simulink model "PV_battery"  (R2017b)
settings: Solver=FixedStepDiscrete  StartTime=0.0  StopTime=1  FixedStep=Ts  RelTol=1e-3
InitFcn:
  | Ts=0.000001;
undefined symbols (not defined in the file): DiscIntNeverNeededParam, Ion, Lithium, sigbuilder_block
libraries: powerlib x29, powerlib_meascontrol x2, simulink x2, fuzblock x1, electricdrivelib x1, re_lib x1
settings Model: Creator=Aria  LastModifiedBy=Asus
settings CodeAppCC: StateflowObjectComments=on
settings SimscapeCC: SimscapeNormalizeSystem=off

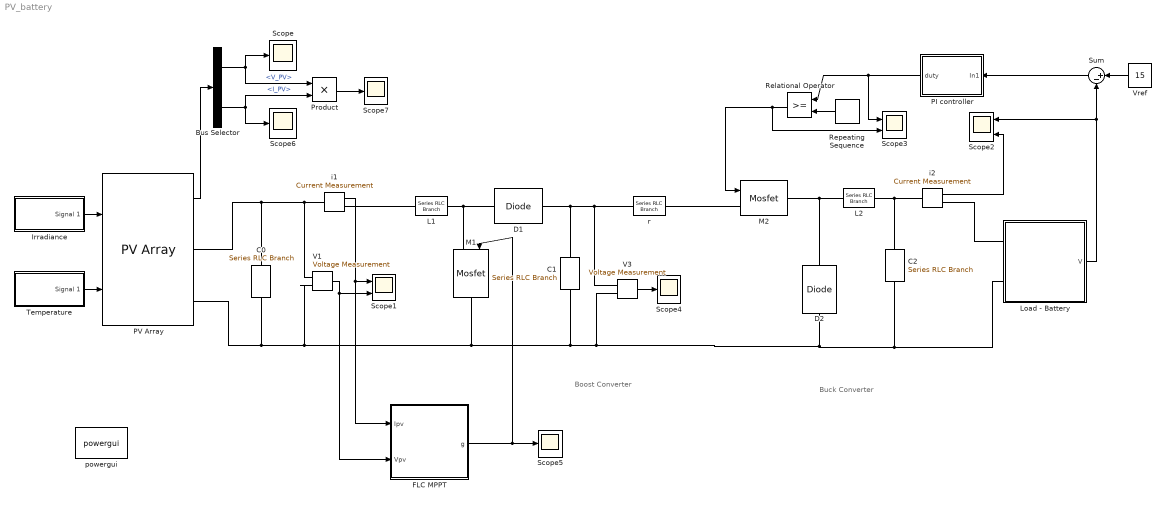
== system PV_battery ==
  note: Buck Converter
  note: Boost Converter
  Bus Selector : BusSelector  OutputSignals=V_PV,I_PV
  C0 : powerlib/Elements/Series RLC Branch  LConnTagsString=__new0  RConnTagsString=__new0  BranchType=C  Resistance=1  Inductance=1e-3  SetiL0=off  InitialCurrent=0  Capacitance=1000e-6  Setx0=off  InitialVoltage=0  Measurements=None
  C1 : powerlib/Elements/Series RLC Branch  LConnTagsString=__new0  RConnTagsString=__new0  BranchType=C  Resistance=1  Inductance=1e-3  SetiL0=off  InitialCurrent=0  Capacitance=0.6e-3  Setx0=off  InitialVoltage=0  Measurements=None
  C2 : powerlib/Elements/Series RLC Branch  LConnTagsString=__new0  RConnTagsString=__new0  BranchType=C  Resistance=1  Inductance=1e-3  SetiL0=off  InitialCurrent=0  Capacitance=140e-6  Setx0=off  InitialVoltage=0  Measurements=None
  D1 : powerlib/Power Electronics/Diode  Ron=0.001  Lon=0  Vf=0.8  IC=0  UseSnubber=off  Rs=100  Cs=500e-09  Measurements=off
  D2 : powerlib/Power Electronics/Diode  Ron=0.001  Lon=0  Vf=0.8  IC=0  UseSnubber=off  Rs=100  Cs=500e-09  Measurements=off
  FLC MPPT : Subsystem
  Irradiance : Subsystem  Tag=STV Subsys  LoadFcn=sigbuilder_block('load');  StartFcn=sigbuilder_block('start');  StopFcn=sigbuilder_block('stop');  ClipboardFcn=sigbuilder_block('clipboard');  mask(Sigbuilder block){tuvar=[0:10]}
      mask help: Simulink:masks:SigbuilderBlock_MD
      mask init:
      | if ~strcmp(get_param(bdroot(gcbh),'SimulationStatus'),'stopped') tuvar = sigbuilder_block('maskInit'); end
      settings: CopyFcn=sigbuilder_block('copy');  DeleteFcn=sigbuilder_block('delete');  ModelCloseFcn=sigbuilder_block('modelClose');  PreSaveFcn=sigbuilder_block('preSave');  PauseFcn=sigbuilder_block('pause');  ContinueFcn=sigbuilder_block('continue');  NameChangeFcn=sigbuilder_block('namechange');  OpenFcn=sigbuilder_block('open',[129.75 81.75 727.5 409.5 ]);  CloseFcn=sigbuilder_block('close');
      mask Display: plot(0, 0, 100, 100,[2, 2, 32, 32, 2], [68, 8, 8, 68, 68],[32, 2], [38, 38], [32, 19, 2],[53, 60, 44], [32, 17, 17, 2],[16, 16, 31, 31]);txt = getActiveGroup(gcbh);text(2, 100, txt,'verticalAlignment', 'top');
  L1 : powerlib/Elements/Series RLC Branch  LConnTagsString=__new0  RConnTagsString=__new0  BranchType=L  Resistance=1  Inductance=0.5e-3  SetiL0=off  InitialCurrent=0  Capacitance=1e-6  Setx0=off  InitialVoltage=0  Measurements=None
  L2 : powerlib/Elements/Series RLC Branch  LConnTagsString=__new0  RConnTagsString=__new0  BranchType=L  Resistance=1  Inductance=20e-3  SetiL0=off  InitialCurrent=0  Capacitance=1e-6  Setx0=off  InitialVoltage=0  Measurements=None
  Load - Battery : Subsystem
  M1 : powerlib/Power Electronics/Mosfet  Ron=0.1  Lon=0  Rd=0.01  Vfd=0  IC=0  Rs=1e5  Cs=inf  Measurements=off
  M2 : powerlib/Power Electronics/Mosfet  Ron=0.1  Lon=0  Rd=0.01  Vfd=0  IC=0  Rs=1e5  Cs=inf  Measurements=off
  PI controller : Subsystem
  PV Array : re_lib/Solar/PV Array  Npar=1  Nser=1  PlotType=one module @ 25 deg.C & specified irradiances  S_vec="[ 1000 800 600  400 ]"  Temp_C_vec="[ 45 25  ]"  ModuleName=Jinzhou Jinmao Photovoltaic Technology JMPV-5M-36-85  PlotWhenSelected=off  Pm=84.9446  Ncell=36  Voc=22  Isc=5.08  Vm=17.66  Im=4.81  beta_Voc_pc=-0.41641  alpha_Isc_pc=0.037008  beta_Voc=-0.09161  alpha_Isc=0.00188  IL=5.102  I0=1.0231e-09  nI=1.0654  Rsh=1144.3491  Rs=0.31769  BAL=off  Tc=1e-6  Tfilter=5e-5
  Product : Product
  Relational Operator : RelationalOperator  OutDataTypeStr=boolean  RndMeth=Simplest
  Repeating Sequence : simulink/Sources/Repeating Sequence  rep_seq_t=[0 0.0002]  rep_seq_y=[0 1]
  Scope{,4..7} (5 alike) : Scope
  Scope1 : Scope  NumInputPorts=2
  Scope2 : Scope  NumInputPorts=2
  Scope3 : Scope  NumInputPorts=2
  Sum : Sum  Inputs=|+-
  Temperature : Subsystem  Tag=STV Subsys  LoadFcn=sigbuilder_block('load');  StartFcn=sigbuilder_block('start');  StopFcn=sigbuilder_block('stop');  ClipboardFcn=sigbuilder_block('clipboard');  mask(Sigbuilder block){tuvar=[0:10]}
      mask help: Simulink:masks:SigbuilderBlock_MD
      mask init:
      | if ~strcmp(get_param(bdroot(gcbh),'SimulationStatus'),'stopped') tuvar = sigbuilder_block('maskInit'); end
      settings: CopyFcn=sigbuilder_block('copy');  DeleteFcn=sigbuilder_block('delete');  ModelCloseFcn=sigbuilder_block('modelClose');  PreSaveFcn=sigbuilder_block('preSave');  PauseFcn=sigbuilder_block('pause');  ContinueFcn=sigbuilder_block('continue');  NameChangeFcn=sigbuilder_block('namechange');  OpenFcn=sigbuilder_block('open',[149.25 143.25 550.5 359.25 ]);  CloseFcn=sigbuilder_block('close');
      mask Display: plot(0, 0, 100, 100,[2, 2, 32, 32, 2], [68, 8, 8, 68, 68],[32, 2], [38, 38], [32, 19, 2],[53, 60, 44], [32, 17, 17, 2],[16, 16, 31, 31]);txt = getActiveGroup(gcbh);text(2, 100, txt,'verticalAlignment', 'top');
  V1 : powerlib/Measurements/Voltage Measurement  PhasorSimulation=off  OutputType=Complex  PSBequivalent=0
  V3 : powerlib/Measurements/Voltage Measurement  PhasorSimulation=off  OutputType=Complex  PSBequivalent=0
  Vref : Constant  Value=15
  i1 : powerlib/Measurements/Current Measurement  PhasorSimulation=off  OutputType=Complex  PSBequivalent=0
  i2 : powerlib/Measurements/Current Measurement  PhasorSimulation=off  OutputType=Complex  PSBequivalent=0
  powergui : powerlib/powergui  Priority=1  SimulationMode=Discrete  SampleTime=Ts  frequency=60  Iterations=50  frequencyindice=0  Pbase=100e6  ErrMax=1e-4  UnitsV=kV  UnitsW=MW  buscounter=0  FunctionMessages=off  echomessages=off  EnableUseOfTLC=off  CurrentSourceSwitches=off  DisableSnubberDevices=off  DisableRonSwitches=off  DisableVfSwitches=off  DisplayEquations=off  SolverType=Tustin/Backward Euler (TBE)  Interpol=off  ExternalGateDelay=off  methode=off  Ts=10  x0status=blocks  SPID=off  SwTol=0  HookPort=off  RestoreLinks=warning  ResistiveCurrentMeasurement=off  Frange=[0:2:500]  Ylog=off  Xlog=on  ShowGrid=off  save=off  variable=ZData  structure=0  ZoomFFT=off  StartTime=0.0  cycles=1  DisplayStyle=1  fundamental=60  FreqAxis=off  MaxFrequency=1000  frequencyindicesteady=1  RmsSteady=1  display=off
  r : powerlib/Elements/Series RLC Branch  LConnTagsString=__new0  RConnTagsString=__new0  BranchType=R  Resistance=1  Inductance=1e-3  SetiL0=off  InitialCurrent=0  Capacitance=1e-6  Setx0=off  InitialVoltage=0  Measurements=None
  wires:
  Irradiance/1(Signal 1) -> PV Array/1
  Temperature/1(Signal 1) -> PV Array/2
  Bus Selector/1 -> Product/1, Scope/1  "<V_PV>"
  Bus Selector/2 -> Scope6/1, Product/2  "<I_PV>"
  Repeating Sequence/1 -> Relational Operator/2
  Relational Operator/1 -> Scope3/2, M2/1
  V3/1 -> Scope4/1
  FLC MPPT/1(g) -> M1/1, Scope5/1
  PI controller/1(duty) -> Scope3/1, Relational Operator/1
  V1/1 -> Scope1/2, FLC MPPT/2(Vpv)
  i1/1 -> FLC MPPT/1(Ipv), Scope1/1
  PV Array/1 -> Bus Selector/1
  Sum/1 -> PI controller/1(In1)
  Vref/1 -> Sum/1
  Load - Battery/1(V) -> Scope2/1, Sum/2
  i2/1 -> Scope2/2
  Product/1 -> Scope7/1
  connections:
  i1/LConn1 -- V1/LConn1 -- C0/LConn1 -- PV Array/RConn1
  D1/LConn1 -- L1/RConn1 -- M1/LConn1
  V3/LConn1 -- r/LConn1 -- C1/LConn1 -- D1/RConn1
  M2/RConn1 -- L2/LConn1 -- D2/RConn1
  i2/LConn1 -- C2/LConn1 -- L2/RConn1
  PV Array/RConn2 -- V1/LConn2 -- Load - Battery/LConn2 -- C2/RConn1 -- D2/LConn1 -- V3/LConn2 -- C1/RConn1 -- M1/RConn1 -- C0/RConn1
  i1/RConn1 -- L1/LConn1
  M2/LConn1 -- r/RConn1
  i2/RConn1 -- Load - Battery/LConn1

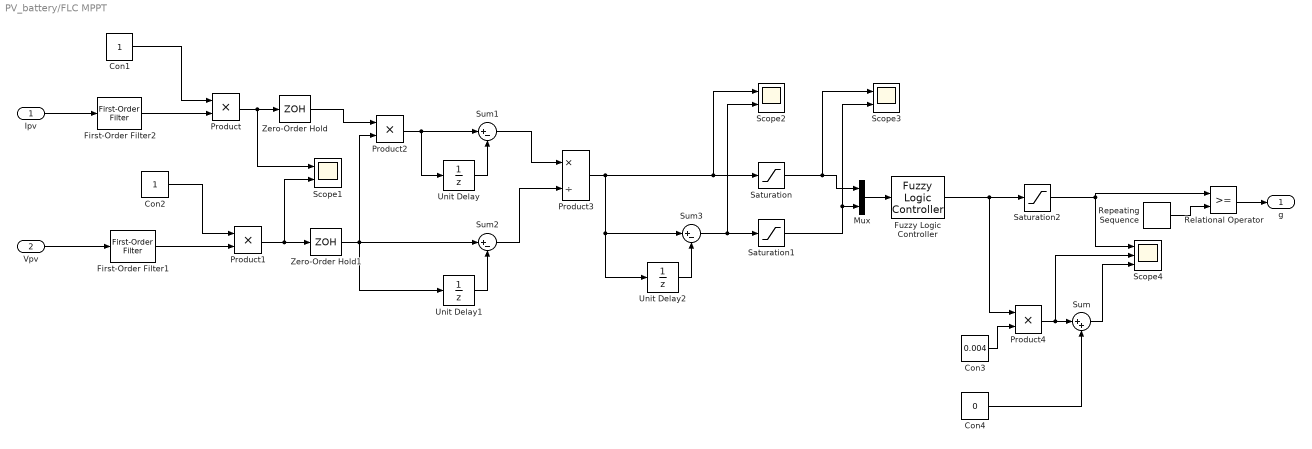
== system PV_battery/FLC MPPT ==
  Ipv : Inport
  Vpv : Inport  Port=2
  Con1 : Constant
  Con2 : Constant
  Con3 : Constant  Value=0.004
  Con4 : Constant  Value=0
  First-Order Filter1 : powerlib_meascontrol/Filters/First-Order Filter  FilterType=Lowpass  Tc=2e-3  Ts=Ts  Initialize=on  Vac_Init=[0, 0, 60]  Vdc_Init=0  PlotResponse=off  FreqRange="[0,  500,  1]"
      settings: SourceProductName=Simscape Power Systems
  First-Order Filter2 : powerlib_meascontrol/Filters/First-Order Filter  FilterType=Lowpass  Tc=5e-3  Ts=Ts  Initialize=on  Vac_Init=[0, 0, 60]  Vdc_Init=0  PlotResponse=off  FreqRange="[0,  500,  1]"
      settings: SourceProductName=Simscape Power Systems
  Fuzzy Logic Controller : fuzblock/Fuzzy Logic  Controller  FIS='PVB.fis'  OutputSampleNumber=101  DataType=double  FuzzifiedInputs=off  RuleFiringStrengths=off  RuleOutputs=off  AggregatedOutputs=off  SimulateUsing=Interpreted execution
  Mux : Mux  Inputs=2
  Product{,1..2,4} (4 alike) : Product
  Product3 : Product  Inputs=*/
  Relational Operator : RelationalOperator  OutDataTypeStr=boolean  RndMeth=Simplest
  Repeating Sequence : simulink/Sources/Repeating Sequence  rep_seq_t=[0 0.0002]  rep_seq_y=[0 1]
  Saturation : Saturate  UpperLimit=10  LowerLimit=-12
  Saturation1 : Saturate  UpperLimit=2  LowerLimit=-2
  Saturation2 : Saturate  UpperLimit=0.41  LowerLimit=0.39
  Scope1 : Scope  NumInputPorts=2
  Scope2 : Scope  NumInputPorts=2
  Scope3 : Scope  NumInputPorts=2
  Scope4 : Scope  NumInputPorts=3
  Sum : Sum  Inputs=|++
  Sum1 : Sum  Inputs=|+-
  Sum2 : Sum  Inputs=|+-
  Sum3 : Sum  Inputs=|+-
  Unit Delay : UnitDelay  SampleTime=-1
  Unit Delay1 : UnitDelay  SampleTime=-1
  Unit Delay2 : UnitDelay  SampleTime=-1
  Zero-Order Hold : ZeroOrderHold  SampleTime=0.0001
  Zero-Order Hold1 : ZeroOrderHold  SampleTime=0.0001
  g : Outport
  wires:
  Sum/1 -> Scope4/3
  First-Order Filter2/1 -> Product/2
  Product1/1 -> Scope1/2, Zero-Order Hold1/1
  Con2/1 -> Product1/1
  Product/1 -> Scope1/1, Zero-Order Hold/1
  Ipv/1 -> First-Order Filter2/1
  Con1/1 -> Product/1
  Vpv/1 -> First-Order Filter1/1
  Zero-Order Hold/1 -> Product2/1
  First-Order Filter1/1 -> Product1/2
  Saturation/1 -> Scope3/1, Mux/1
  Sum2/1 -> Product3/2
  Sum1/1 -> Product3/1
  Sum3/1 -> Scope2/2, Saturation1/1
  Product2/1 -> Unit Delay/1, Sum1/1
  Con4/1 -> Sum/2
  Con3/1 -> Product4/2
  Saturation1/1 -> Scope3/2, Mux/2
  Mux/1 -> Fuzzy Logic Controller/1
  Product4/1 -> Scope4/2, Sum/1
  Fuzzy Logic Controller/1 -> Saturation2/1, Product4/1
  Unit Delay/1 -> Sum1/2
  Zero-Order Hold1/1 -> Sum2/1, Unit Delay1/1, Product2/2
  Unit Delay1/1 -> Sum2/2
  Product3/1 -> Scope2/1, Saturation/1, Sum3/1, Unit Delay2/1
  Unit Delay2/1 -> Sum3/2
  Saturation2/1 -> Relational Operator/1, Scope4/1
  Repeating Sequence/1 -> Relational Operator/2
  Relational Operator/1 -> g/1

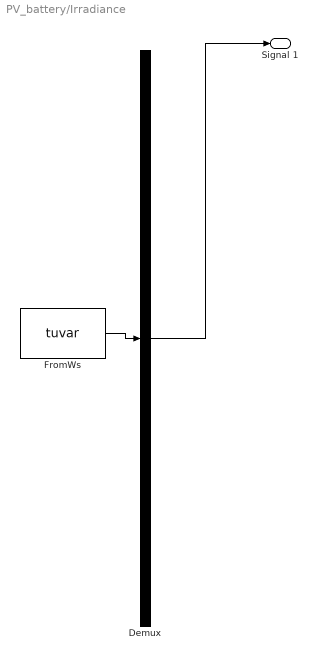
== system PV_battery/Irradiance ==
  Demux : Demux  Tag=STV Demux  Outputs=1
  FromWs : FromWorkspace  Tag=STV FromWs  VariableName=tuvar  SampleTime=0
      SigBuilderData=|
      | common.afterFinalStr = 'Extrapolate'
      | common.sampleTime = 0
      | dataSet.timeRange = [0 1]
      | dataSet.name = 'Group 1'
      | sbobj.Groups.Name = 'Group 1'
      | sbobj.Groups.Signals.Name = 'Signal 1'
      | sbobj.Groups.Signals.XData = [0 0.2 0.2 0.4 0.4 0.6 0.6 1]
      | sbobj.Groups.Signals.YData = [1000 1000 700 700 1000 1000 700 700]
      | sbobj.Groups.TimeRange = [0 1]
  Signal 1 : Outport  Tag=STV Outport
  wires:
  Demux/1 -> Signal 1/1
  FromWs/1 -> Demux/1

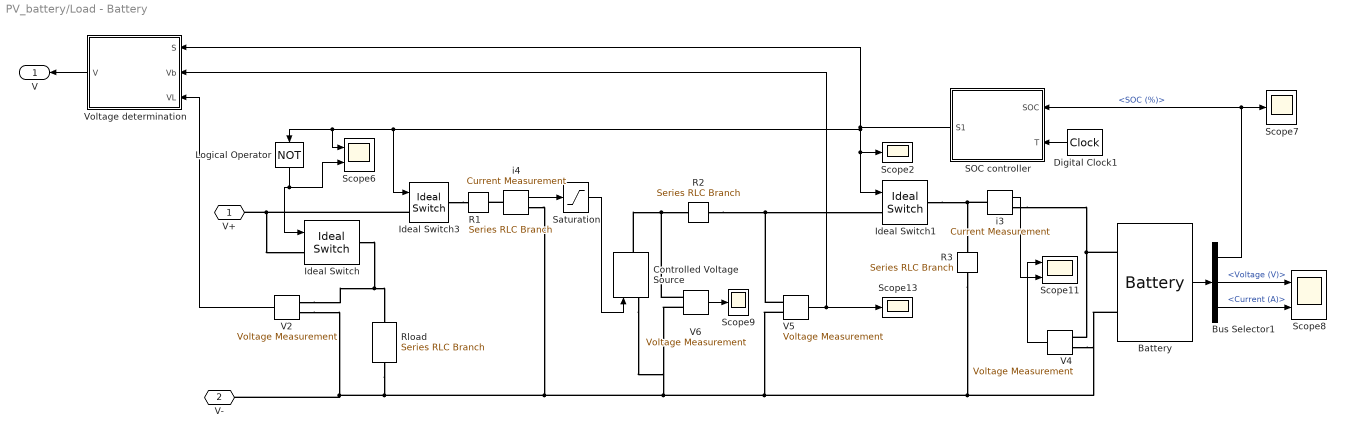
== system PV_battery/Load - Battery ==
  Battery : electricdrivelib/Extra Sources/Battery  BatType=Lithium-Ion  ShowTempParam=off  ThermalPreset=no  ShowAgeParam=off  NomV=15  NomQ=2  SOC=50  Batt_Tr=15  PresetModel=on  MaxQ=2  MinV=11.25  FullV=17.4598  Dis_rate=0.86957  R=0.075  Normal_OP=1.8087  expZone="[16.2058    0.0982609]"  current="[2  5  8]"  Units=Time  Tci=20  NomT=25  T2=0  MaxQ2=2.208  FullV2=3.45  Normal_OP2=2.8  expZone2="[3.22        0.23]"  Rca=0.6  ti=1000  Dp=0  Neq0=0  Tsim=1e6  Ta1=25  Qeol=5.4*0.9  Reol=0.013333*1.2  Char_age=[2.3478, 3]  Dis_age=[2.3478, 10]  N1=1500  N2=10500  N3=1000  N4=1400  Ta2=45  N5=950
  Bus Selector1 : BusSelector  OutputSignals=SOC (%),Voltage (V),Current (A)
  Controlled Voltage Source : powerlib/Electrical Sources/Controlled Voltage Source  Initialize=on  Source_Type=AC  Amplitude=0  Phase=0  Frequency=0  Measurements=None
  Digital Clock1 : DigitalClock  SampleTime=0.001
  Ideal Switch : powerlib/Power Electronics/Ideal Switch  Ron=0.001  Lon=0  IC=0  Rs=1e5  Cs=inf  Measurements=off
  Ideal Switch1 : powerlib/Power Electronics/Ideal Switch  Ron=0.001  Lon=0  IC=0  Rs=1e5  Cs=inf  Measurements=off
  Ideal Switch3 : powerlib/Power Electronics/Ideal Switch  Ron=0.001  Lon=0  IC=0  Rs=1e5  Cs=inf  Measurements=off
  Logical Operator : Logic  Operator=NOT  AllPortsSameDT=off  OutDataTypeStr=boolean
  R1 : powerlib/Elements/Series RLC Branch  LConnTagsString=__new0  RConnTagsString=__new0  BranchType=R  Resistance=8  Inductance=2  SetiL0=off  InitialCurrent=0  Capacitance=1e-6  Setx0=off  InitialVoltage=0  Measurements=None
  R2 : powerlib/Elements/Series RLC Branch  LConnTagsString=__new0  RConnTagsString=__new0  BranchType=R  Resistance=1.5  Inductance=2  SetiL0=off  InitialCurrent=0  Capacitance=1e-6  Setx0=off  InitialVoltage=0  Measurements=None
  R3 : powerlib/Elements/Series RLC Branch  LConnTagsString=__new0  RConnTagsString=__new0  BranchType=R  Resistance=30  Inductance=2  SetiL0=off  InitialCurrent=0  Capacitance=1e-6  Setx0=off  InitialVoltage=0  Measurements=None
  Rload : powerlib/Elements/Series RLC Branch  LConnTagsString=__new0  RConnTagsString=__new0  BranchType=R  Resistance=5  Inductance=2  SetiL0=off  InitialCurrent=0  Capacitance=1e-6  Setx0=off  InitialVoltage=0  Measurements=None
  SOC controller : MATLAB Function  TreatAsAtomicUnit=on
  Saturation : Saturate  UpperLimit=2  LowerLimit=0
  Scope11 : Scope  NumInputPorts=2
  Scope{2,7,9,13} (4 alike) : Scope
  Scope6 : Scope  NumInputPorts=2
  Scope8 : Scope  NumInputPorts=2
  V{2,4..6} (4 alike) : powerlib/Measurements/Voltage Measurement  PhasorSimulation=off  OutputType=Complex  PSBequivalent=0
  Voltage determination : MATLAB Function  TreatAsAtomicUnit=on
  i3 : powerlib/Measurements/Current Measurement  PhasorSimulation=off  OutputType=Complex  PSBequivalent=0
  i4 : powerlib/Measurements/Current Measurement  PhasorSimulation=off  OutputType=Complex  PSBequivalent=0
  V+ : PMIOPort  Port=1  Side=Left
  V- : PMIOPort  Port=2  Side=Left
  V : Outport
  wires:
  i4/1 -> Saturation/1
  V5/1 -> Voltage determination/2(Vb), Scope13/1
  Digital Clock1/1 -> SOC controller/2(T)
  Bus Selector1/1 -> SOC controller/1(SOC), Scope7/1  "<SOC (%)>"
  Battery/1 -> Bus Selector1/1
  Bus Selector1/2 -> Scope8/1  "<Voltage (V)>"
  Bus Selector1/3 -> Scope8/2  "<Current (A)>"
  Logical Operator/1 -> Ideal Switch/1, Scope6/2
  V2/1 -> Voltage determination/3(VL)
  i3/1 -> Scope11/2
  V4/1 -> Scope11/1
  SOC controller/1(S1) -> Scope6/1, Logical Operator/1, Ideal Switch3/1, Scope2/1, Ideal Switch1/1, Voltage determination/1(S)
  Saturation/1 -> Controlled Voltage Source/1
  V6/1 -> Scope9/1
  Voltage determination/1(V) -> V/1
  connections:
  Controlled Voltage Source/RConn1 -- V6/LConn1 -- R2/LConn1
  R2/RConn1 -- V5/LConn1 -- Ideal Switch1/LConn1
  Ideal Switch1/RConn1 -- R3/RConn1 -- i3/LConn1
  Rload/LConn1 -- V-/RConn1 -- V2/LConn2 -- R3/LConn1 -- Battery/LConn2 -- V4/LConn2 -- V5/LConn2 -- V6/LConn2 -- Controlled Voltage Source/LConn1 -- i4/RConn1
  Ideal Switch3/LConn1 -- Ideal Switch/LConn1 -- V+/RConn1
  Ideal Switch/RConn1 -- Rload/RConn1 -- V2/LConn1
  i3/RConn1 -- Battery/LConn1 -- V4/LConn1
  i4/LConn1 -- R1/RConn1
  Ideal Switch3/RConn1 -- R1/LConn1

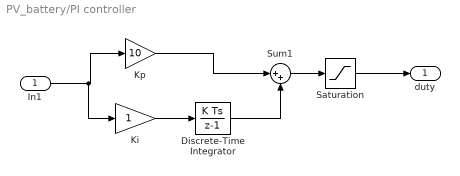
== system PV_battery/PI controller ==
  In1 : Inport
  Discrete-Time Integrator : DiscreteIntegrator  InitialConditionSetting=State (most efficient)  SampleTime=Ts  ICPrevOutput=DiscIntNeverNeededParam  ICPrevScaledInput=DiscIntNeverNeededParam
  Ki : Gain
  Kp : Gain  Gain=10
  Saturation : Saturate  UpperLimit=0.7  LowerLimit=0.5
  Sum1 : Sum  Inputs=|++
  duty : Outport
  wires:
  Sum1/1 -> Saturation/1
  Discrete-Time Integrator/1 -> Sum1/2
  Ki/1 -> Discrete-Time Integrator/1
  Kp/1 -> Sum1/1
  In1/1 -> Ki/1, Kp/1
  Saturation/1 -> duty/1

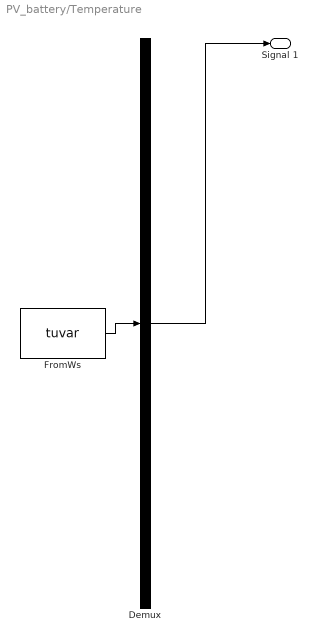
== system PV_battery/Temperature ==
  Demux : Demux  Tag=STV Demux  Outputs=1
  FromWs : FromWorkspace  Tag=STV FromWs  VariableName=tuvar  SampleTime=0
      SigBuilderData=|
      | common.afterFinalStr = 'Extrapolate'
      | common.sampleTime = 0
      | dataSet.timeRange = [0 1]
      | dataSet.name = 'Group 1'
      | sbobj.Groups.Name = 'Group 1'
      | sbobj.Groups.Signals.Name = 'Signal 1'
      | sbobj.Groups.Signals.XData = [0 0.4 0.4 1]
      | sbobj.Groups.Signals.YData = [25 25 60 60]
      | sbobj.Groups.TimeRange = [0 1]
  Signal 1 : Outport  Tag=STV Outport
  wires:
  Demux/1 -> Signal 1/1
  FromWs/1 -> Demux/1

== matlab function PV_battery/Load - Battery/Voltage determination ==
  data: S input; V output; Vb input; VL input
function V = fcn1(S,Vb,VL)
persistent a

     if S==1
        a=Vb;
     else
        a=VL;
     end
V=a;
end

== matlab function PV_battery/Load - Battery/SOC controller ==
  data: SOC input; S1 output; T input
function S1  = fcn(SOC,T)
persistent a n

if isempty(a)
    a=0;
end
if isempty(n) 
    n=0;  
end
if (T>n*0.00001) % sample time is 0.00001s
    n=n+1;
     if SOC>35 && SOC<80
       a=1;     
     else
       a=0;

     end
end
S1 = a;
end
